simulink model "NewtTriggerVanDerPol"  (R2023a)
settings: Solver=ode45  StartTime=0  StopTime=1000  FixedStep=1e-4  RelTol=1e-4  AbsTol=1e-5
values from neighbouring files (symbols this model uses):
  A = [0 1;-1 -1]    [runVanDerPolTrigger.m]
  Ar = A    [runVanDerPolTrigger.m]
  B = params.B    [plotSimulinkResults.m]    (also in runVanDerPolTrigger.m = [0;1])
  Br = B    [runVanDerPolTrigger.m]
  centers = gCenters    [runVanDerPolTrigger.m]
  del = 0    [runVanDerPolTrigger.m]
  epsilon = PowerBound*R+delta    [runVanDerPolTrigger.m]
  gf = 1e4    (= 10000)    [runVanDerPolTrigger.m]
  K = real(kermat(centers,centers,type,par,scale))    [runVanDerPolTrigger.m]
  kx = place(A,B,pDes)    [runVanDerPolTrigger.m]
  lambda0 = lambda(end,:)'    [runVanDerPolTrigger.m]
  mu = 3    [runVanDerPolTrigger.m]
  noisy = true    [runVanDerPolTrigger.m]
  norm_f = max(norm_fs(condT < 1e12))    [runVanDerPolTrigger.m]
  P = params.P    [plotSimulinkResults.m]    (also in runVanDerPolTrigger.m = sqrt(z(jj+2)-w(jj+2)))
  par = 6    [runVanDerPolTrigger.m]
  rmax = params.rmax    [plotSimulinkResults.m]    (also in runVanDerPolTrigger.m = norm(xr0))
  Ro = 2*sqrt(2)+0.3    [runVanDerPolTrigger.m]
  scale = 0.3    [runVanDerPolTrigger.m]
  tol = C*PowerBound*R    [runVanDerPolTrigger.m]
  triggered = 0    [runVanDerPolTrigger.m]
  Tswitch_min = 5    [runVanDerPolTrigger.m]
  V = zeros(N,N)    [runVanDerPolTrigger.m]
  x0 = x(end,:)    [runVanDerPolTrigger.m]
  xr0 = xr(end,:)    [runVanDerPolTrigger.m]
settings Model: Creator=owned  LastModifiedBy=Ownedpilot
settings SolverCC: AlgebraicLoopSolver=TrustRegion
settings OptimizationCC: ReuseModelBlockBuffer=off
settings DebuggingCC: UnconnectedInputMsg=warning  UnconnectedOutputMsg=warning  UnconnectedLineMsg=warning
settings ModelReferenceCC: EnableRefExpFcnMdlSchedulingChecks=on
settings RTWCC: DLArmComputeVersion=19.05

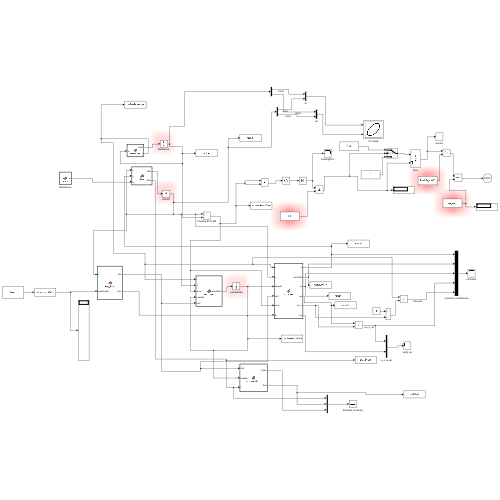
[thumbnail: Simulink's stored preview of the top-level diagram]
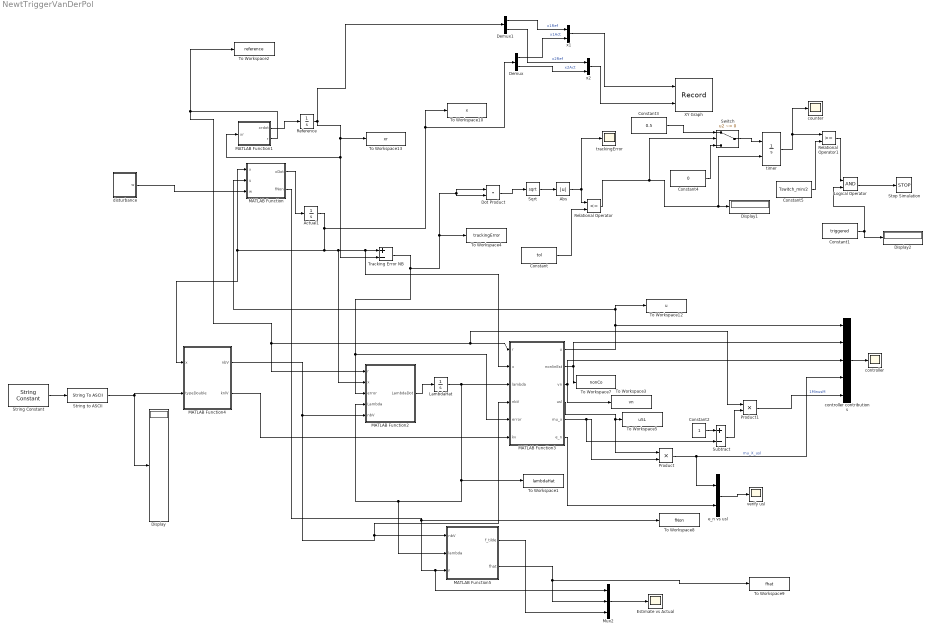
== system NewtTriggerVanDerPol ==
  Abs : Abs  SaturateOnIntegerOverflow=off
  Actual1 : Integrator  InitialCondition=x0
  Constant : Constant  Value=tol
  Constant1 : Constant  Value=triggered
  Constant2 : Constant
  Constant3 : Constant  Value=0.5
  Constant4 : Constant  Value=0
  Constant5 : Constant  Value=Tswitch_min/2
  Demux : Demux  Outputs=2
  Demux1 : Demux  Outputs=2
  Display : Display
  Display1 : Display
  Display2 : Display
  Dot Product : DotProduct  OutDataTypeStr=Inherit: Inherit via internal rule
  Estimate vs Actual : Scope
  LambdaHat : Integrator  InitialCondition=lambda0
  Logical Operator : Logic  AllPortsSameDT=off  OutDataTypeStr=boolean
  MATLAB Function : MATLAB Function  TreatAsAtomicUnit=on
  MATLAB Function1 : MATLAB Function  TreatAsAtomicUnit=on
  MATLAB Function2 : MATLAB Function  TreatAsAtomicUnit=on
  MATLAB Function3 : MATLAB Function  TreatAsAtomicUnit=on
  MATLAB Function4 : MATLAB Function  TreatAsAtomicUnit=on
  MATLAB Function5 : MATLAB Function  TreatAsAtomicUnit=on
  Mux2 : Mux  Inputs=3
  Product : Product
  Product1 : Product
  Reference : Integrator  InitialCondition=xr0
  Relational Operator : RelationalOperator  Operator=<=  OutDataTypeStr=boolean  RndMeth=Simplest  InputSameDT=off
  Relational Operator1 : RelationalOperator  OutDataTypeStr=boolean  RndMeth=Simplest  InputSameDT=off
  Sqrt : Sqrt
  Stop Simulation : Stop
  String Constant : StringConstant  String=type
  String to ASCII : StringToASCII
  Subtract : Sum  Inputs=+-
  Switch : Switch  Criteria=u2 ~= 0  SaturateOnIntegerOverflow=off  InputSameDT=off
  To Workspace1 : ToWorkspace  VariableName=lambdaHat  SaveFormat=Timeseries  SampleTime=-1
  To Workspace10 : ToWorkspace  VariableName=x  SaveFormat=Timeseries  SampleTime=-1
  To Workspace12 : ToWorkspace  VariableName=u  SaveFormat=Timeseries  SampleTime=-1
  To Workspace13 : ToWorkspace  VariableName=xr  SaveFormat=Timeseries  SampleTime=-1
  To Workspace2 : ToWorkspace  VariableName=reference  SaveFormat=Timeseries  SampleTime=-1
  To Workspace3 : ToWorkspace  VariableName=vn  SaveFormat=Timeseries  SampleTime=-1
  To Workspace4 : ToWorkspace  VariableName=trackingError  SaveFormat=Timeseries  SampleTime=-1
  To Workspace5 : ToWorkspace  VariableName=uSL  SaveFormat=Timeseries  SampleTime=-1
  To Workspace7 : ToWorkspace  VariableName=nonCo  SaveFormat=Timeseries  SampleTime=-1
  To Workspace8 : ToWorkspace  VariableName=fNon  SaveFormat=Timeseries  SampleTime=-1
  To Workspace9 : ToWorkspace  VariableName=fhat  SaveFormat=Timeseries  SampleTime=-1
  Tracking Error NB : Sum  Inputs=+-
  XY Graph : Record  FileSettingsInternal="{\"entries\":[{\"content\":{\"excelSettings\":{\"content\":{},\"type\":\"Streamout.ExcelSettings\"}},\"type\":\"Streamout.FileSettingStorage\",\"uuid\":\"\"}],\"packageUris\":[\"http:\\/\\/schema.mathworks.com\\/mf0\\/streamout_blocks\\/R2020a\"],\"version\":\"1.0\"}"  Layout=[1 1]  SignalsInternal="{\"entries\":[{\"content\":{\"signals\":[{\"content\":{\"blockPath\":[],\"dimensions\":[2],\"domain\":\"\",\"hasChildren\":true,\"lineColor\":\"#77ac30\",\"port\":1,\"signalID\":25,\"signalName\":\"x1\"},\"type\":\"RecordBlkView.Signal\",\"uuid\":\"\"},{\"content\":{\"blockPath\":[],\"channel\":[1],\"dimensions\":[2],\"domain\":\"\",\"lineColor\":\"#b746ff\",\"parentID\":25,\"plots\":[1],\"port\":1,\"signalID\":26,\"signalName\":\"x1\"},\"type\":\"RecordBlkView.Signal\",\"uuid\":\"\"},{\"content\":{\"blockPath\":[],\"channel\":[2],\"dimensions\":[2],\"domain\":\"\",\"lineColor\":\"#64d413\",\"parentID\":25,\"plots\":[1],\"port\":1,\"signalID\":27,\"signalName\":\"x1\"},\"type\":\"RecordBlkView.Signal\",\"uuid\":\"\"},{\"content\":{\"blockPath\":[],\"dimensions\":[2],\"domain\":\"\",\"hasChildren\":true,\"lineColor\":\"#a2142f\",\"port\":2,\"signalID\":32,\"signalName\":\"x2\"},\"type\":\"RecordBlkView.Signal\",\"uuid\":\"\"},{\"content\":{\"blockPath\":[],\"channel\":[1],\"dimensions\":[2],\"domain\":\"\",\"lineColor\":\"#0072bd\",\"parentID\":32,\"plots\":[1],\"port\":2,\"signalID\":33,\"signalName\":\"x2\"},\"type\":\"RecordBlkView.Signal\",\"uuid\":\"\"},{\"content\":{\"blockPath\":[],\"channel\":[2],\"dimensions\":[2],\"domain\":\"\",\"lineColor\":\"#ff13a6\",\"parentID\":32,\"plots\":[1],\"port\":2,\"signalID\":34,\"signalName\":\"x2\"},\"type\":\"RecordBlkView.Signal\",\"uuid\":\"\"}]},\"type\":\"RecordBlkView.InputSignals\",\"uuid\":\"\"}],\"packageUris\":[\"http:\\/\\/schema.mathworks.com\\/mf0\\/streamout_blocks\\/R2020a\"],\"version\":\"1.0\"}"  VisualizationBindings="{\"xyplotplugin\":{\"info\":[{\"series\":[{\"bindingParametersList\":[{\"parameter\":\"X-Axis\",\"signalID\":27,\"signalName\":\"x1(2)\"},{\"parameter\":\"Y-Axis\",\"signalID\":34,\"signalName\":\"x2(2)\"}],\"seriesID\":29538},{\"bindingParametersList\":[{\"parameter\":\"X-Axis\",\"signalID\":26,\"signalName\":\"x1(1)\"},{\"parameter\":\"Y-Axis\",\"signalID\":33,\"signalName\":\"x2(1)\"}],\"seriesID\":30905}],\"subplotID\":1}]}}"  CompatibilityTag=XY
  controller : Scope
  controller contributions : Mux  Inputs=5
  counter : Scope
  disturbance : MATLAB Function  TreatAsAtomicUnit=on
  e_n vs usl : Mux  Inputs=2
  timer : Integrator  ExternalReset=falling
  trackingError : Scope
  verify usl : Scope
  x1 : Mux  Inputs=2
  x2 : Mux  Inputs=2
  wires:
  MATLAB Function1/2(r) -> To Workspace2/1, MATLAB Function2/1(r), Product1/1, MATLAB Function3/1(r)
  MATLAB Function1/1(xrdot) -> Reference/1
  Reference/1 -> Tracking Error NB/2, MATLAB Function1/1(xr), To Workspace13/1, Demux1/1
  MATLAB Function4/1(nbV) -> MATLAB Function5/1(nbV), MATLAB Function3/4(nbV), MATLAB Function2/5(nbV)
  LambdaHat/1 -> MATLAB Function5/2(lambda), MATLAB Function2/4(Lambda), To Workspace1/1, MATLAB Function3/3(lambda)
  String Constant/1 -> String to ASCII/1
  String to ASCII/1 -> Display/1, MATLAB Function4/2(typeDouble)
  Mux2/1 -> Estimate vs Actual/1
  disturbance/1(w) -> MATLAB Function/3(w)
  MATLAB Function2/1(LambdaDot) -> LambdaHat/1
  MATLAB Function/1(xDot) -> Actual1/1
  MATLAB Function5/2(fhat) -> Mux2/2, To Workspace9/1
  MATLAB Function/2(fNon) -> Mux2/1, MATLAB Function5/3(f), To Workspace8/1
  MATLAB Function3/2(nonlinEst) -> To Workspace7/1, controller contributions/2
  Actual1/1 -> Demux/1, To Workspace10/1, MATLAB Function2/2(x), MATLAB Function3/2(x), Tracking Error NB/1, MATLAB Function/1(x), MATLAB Function4/1(x)
  Constant/1 -> Relational Operator/2
  Tracking Error NB/1 -> Dot Product/1, Dot Product/2, To Workspace4/1, MATLAB Function3/5(error), MATLAB Function2/3(error)
  Sqrt/1 -> Abs/1
  Logical Operator/1 -> Stop Simulation/1
  Constant1/1 -> Logical Operator/2, Display2/1
  Dot Product/1 -> Sqrt/1
  Abs/1 -> Relational Operator/1, trackingError/1
  Demux1/1 -> x1/1  "x1Ref"
  Demux/1 -> x1/2  "x1Act"
  Demux1/2 -> x2/1  "x2Ref"
  Demux/2 -> x2/2  "x2Act"
  x1/1 -> XY Graph/1
  x2/1 -> XY Graph/2
  controller contributions/1 -> controller/1
  MATLAB Function4/2(knlV) -> MATLAB Function3/6(kv)
  MATLAB Function3/1(u) -> controller contributions/1, MATLAB Function/2(u), To Workspace12/1
  MATLAB Function3/3(vn) -> To Workspace3/1, controller contributions/3
  MATLAB Function3/6(e_n) -> e_n vs usl/2
  e_n vs usl/1 -> verify usl/1
  MATLAB Function5/1(f_tilde) -> Mux2/3
  MATLAB Function3/4(usl) -> Product/1, To Workspace5/1
  Product/1 -> controller contributions/4, e_n vs usl/1  "mu_X_usl"
  MATLAB Function3/5(mu_x) -> Subtract/2, Product/2
  Constant2/1 -> Subtract/1
  Subtract/1 -> Product1/2
  Product1/1 -> controller contributions/5  "1MinusM"
  Constant5/1 -> Relational Operator1/2
  Relational Operator1/1 -> Logical Operator/1
  timer/1 -> counter/1, Relational Operator1/1
  Relational Operator/1 -> Switch/2, timer/2, Display1/1
  Constant3/1 -> Switch/1
  Switch/1 -> timer/1
  Constant4/1 -> Switch/3

== matlab function NewtTriggerVanDerPol/MATLAB Function3 ==
  data: r input; x input; lambda input size=[N 1]; nbV input size=[N,1]; u output; epsilon parameter; B parameter; nonlinEst output; error input; kv input size=[N,1]; del parameter; P parameter; norm_f parameter; Ro parameter; rmax parameter; kx parameter; vn output; usl output; mu_x output; e_n output
function [u,nonlinEst,vn,usl,mu_x,e_n] = controller(r, x, lambda, nbV,epsilon,B,error,kv, del, P,norm_f,Ro,rmax,kx)
pow_x = real(sqrt(complex(1 - nbV'*nbV)));

e_n = pow_x*norm_f;
%% RKHS smooth switching function

if abs(B'*P*error) > epsilon
    vn = sign(B'*P*error)*e_n;
else
    vn = 1/epsilon*B'*P*error*e_n;
end


%% RKHS Deadzone
% vn = 0;
%% State Limiting
RB = Ro;
mu_x = max([0,min([1,(norm(x)-del*RB)/((1-del)*RB)])]);
ksl = rmax + e_n;
usl =-ksl*sign(B'*P*error);
u =  lambda'*nbV+vn + (1-mu_x)*r +mu_x*usl;

%% Feedback with Desired Poles
% u = -kx*x + r +lambda'*nbV+vn;
nonlinEst = lambda'*nbV;
end

== matlab function NewtTriggerVanDerPol/MATLAB Function4 ==
  data: x input; centers parameter; typeDouble input; nbV output; scale parameter; par parameter; K parameter; V parameter; knlV output
function [nbV,knlV]  = Knl_Eval(x,centers,typeDouble, scale, par,K,V)
    xC = [x(1),x(2)];
    type = char(typeDouble(typeDouble~=0));
    knlV = real(kermat(centers,xC,type,par,scale));
    N = size(centers,1);
    z = diag(K);
    v_x = zeros(N,1);
    P = sqrt(K(1,1));

    v_x(1) = knlV(1)/P;
%     
%     V = zeros(N,N);
%     if N > 1
%         V(:,1) = K(:,1)/P;
%         w = V(:,1).^2;
%         NN = V(2,:)*v_x;
%         P = sqrt(z(2)-w(2));
%         
%         for jj = 1:N-1
%             e = zeros(N,1);
%             e(jj+1) = 1;
%             Vm = V(:,1:jj);
%             u = K*e-Vm*Vm'*e;
%             u_x = knlV(jj+1) - NN;
%             v_x(jj+1) = u_x/P; % Newton Basis evaluated at x
%             V(:,jj+1) = u/P; % Newton Basis evaluated at the centers
%             w = V(:,jj+1).^2 + w; % Updating sum of Newton basis squared at the centers
%             if jj ~=N-1
%                 NN = V(jj+2,:)*v_x;
%                 P = sqrt(z(jj+2)-w(jj+2));
%             end
%         end
%     end
%     nbV = v_x;

    
    if N > 1
        w = V(1:N,1).^2;
        NN = V(2,1:N)*v_x;
        P = sqrt(z(2)-w(2));
        
        for jj = 1:N-1
            u_x = knlV(jj+1) - NN;
            v_x(jj+1) = u_x/P; % Newton Basis evaluated at x
            w = V(1:N,jj+1).^2 + w; % Updating sum of Newton basis squared at the centers
            if jj ~=N-1
                NN = V(jj+2,1:N)*v_x;
                P = sqrt(z(jj+2)-w(jj+2));
            end
        end
    end
    nbV = v_x;


end

== matlab function NewtTriggerVanDerPol/MATLAB Function5 ==
  data: nbV input; f_tilde output; lambda input; fhat output; f input
function [f_tilde,fhat]  = functionError(nbV,lambda,f)
fhat = -lambda'*nbV;
f_tilde = f-fhat;

== matlab function NewtTriggerVanDerPol/disturbance ==
  data: w output; delta parameter
function w   = plant(delta)
% 
w = 0.5*rand;

== matlab function NewtTriggerVanDerPol/MATLAB Function1 ==
  data: xr input; xrdot output; Ar parameter; Br parameter; r output
function [xrdot,r] = reference(xr,Ar, Br)
r = xr(2);
xrv = [xr(1);xr(2)];
xrdot = Ar*xrv+Br*r;

== matlab function NewtTriggerVanDerPol/MATLAB Function ==
  data: x input; u input; A parameter; B parameter; w input; xDot output; fNon output; mu parameter; noisy parameter
function [xDot,fNon]  = plant(x,u,A, B,w,mu,noisy)
% 
% targetKnlV = real(kermat(interps,x,'ms',targetNu-Dim/2,targetScale));
% f = targetCoefs'*targetKnlV;
xv = [x(1);x(2)];

% targetKnlV_NB = real(kermat(interps,xNB,'ms',targetNu-Dim/2,targetScale));
% fNB = targetCoefs'*targetKnlV_NB;
fNon = (1+mu)*x(2)-mu*x(1)^2*x(2);

if noisy
    d_t=[0.1*tanh(x(1)*x(2)) ; 0];
else
    d_t=[0;0];
end

xDot = A*xv+B*(u+fNon)+d_t;

== matlab function NewtTriggerVanDerPol/MATLAB Function2 ==
  data: gf parameter; LambdaDot output; r input; x input; error input; Lambda input; nbV input size=[N,1]; epsilon parameter; P parameter; B parameter
function LambdaDot  = evo_law(gf, r, x, error,  Lambda,  nbV,epsilon,P, B)
sigma = zeros(size(error,1),1);
% for jj = 1:size(error,1)
%     if abs(error(jj)) < epsilon
%         sigma(jj) = error(jj)/epsilon;
%     else
%         sigma(jj) = sign(error(jj));
%     end
% end

%LambdaDot=-double(norm(error,2)>0.7*epsilon)*gf*nbV*B'*P*(error-epsilon*sigma);
LambdaDot=-gf*nbV*B'*P*(error-epsilon*sigma);

end
